simulink subsystem "AirframeActuators"  (R2023b)
settings: Solver=VariableStepAuto  StartTime=0.0  StopTime=10.0  RelTol=1e-3
libraries: aerolibactuator x3
settings Model: Creator=szdaniel  LastModifiedBy=szdaniel

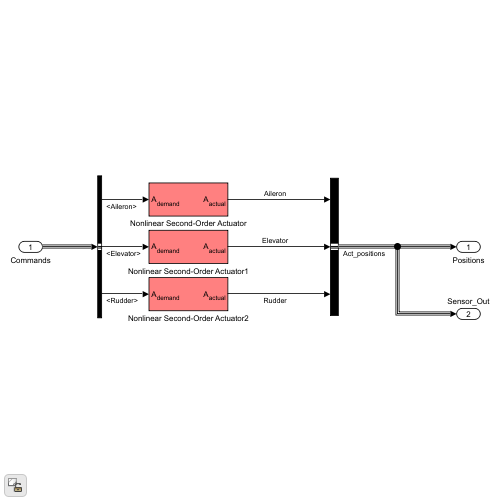
[thumbnail: Simulink's stored preview of the top-level diagram]
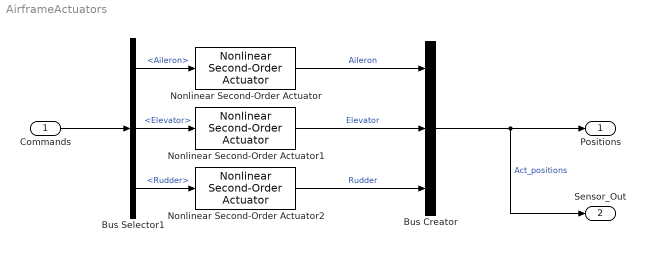
== system AirframeActuators ==
  Commands : Inport
  Bus Creator : BusCreator  Inputs=3
  Bus Selector1 : BusSelector  OutputSignals=Aileron,Elevator,Rudder
  Nonlinear Second-Order Actuator : aerolibactuator/Nonlinear Second-Order Actuator  wn_fin=wn_act  z_fin=z_act  fin_max=maxdef_aileron  fin_min=mindef_aileron  fin_maxrate=Inf  fin_act_0=0  fin_act_vel=0
  Nonlinear Second-Order Actuator1 : aerolibactuator/Nonlinear Second-Order Actuator  wn_fin=wn_act  z_fin=z_act  fin_max=maxdef_elevator  fin_min=mindef_elevator  fin_maxrate=Inf  fin_act_0=0  fin_act_vel=0
  Nonlinear Second-Order Actuator2 : aerolibactuator/Nonlinear Second-Order Actuator  wn_fin=wn_act  z_fin=z_act  fin_max=maxdef_rudder  fin_min=mindef_rudder  fin_maxrate=Inf  fin_act_0=0  fin_act_vel=0
  Positions : Outport  VectorParamsAs1DForOutWhenUnconnected=off
  Sensor_Out : Outport  Port=2  VectorParamsAs1DForOutWhenUnconnected=off
  wires:
  Commands/1 -> Bus Selector1/1
  Bus Selector1/1 -> Nonlinear Second-Order Actuator/1  "<Aileron>"
  Bus Selector1/2 -> Nonlinear Second-Order Actuator1/1  "<Elevator>"
  Bus Selector1/3 -> Nonlinear Second-Order Actuator2/1  "<Rudder>"
  Nonlinear Second-Order Actuator2/1 -> Bus Creator/3  "Rudder"
  Bus Creator/1 -> Positions/1, Sensor_Out/1  "Act_positions"
  Nonlinear Second-Order Actuator/1 -> Bus Creator/1  "Aileron"
  Nonlinear Second-Order Actuator1/1 -> Bus Creator/2  "Elevator"
